simulink model "runsim"  (R2019a)
settings: Solver=VariableStepAuto  StartTime=0.0  StopTime=10.0  RelTol=1e-3
values from neighbouring files (symbols this model uses):
  omega = zeros(N-1,1)    [dubincarminimisevel_venanzio.m]    (also in dubincarminimisevel_venanzio2.m; dubincarminimisevel_venanzio_fine.m; dubincarminimisevel_venanzio_orig.m)
  v = rand(N-1,1)    [DubinsCarMinVel_5varmodel.m]    (also in DubinsCarMinVel_6varmodel.m; DubinsCar_bloatedcode.m = X(:,5); dubincarminimisevel.m = X(:,5); dubincarminimisevel_venanzio.m = ones(N-1,1))
settings Model: Creator=vcichella  LastModifiedBy=Thomas

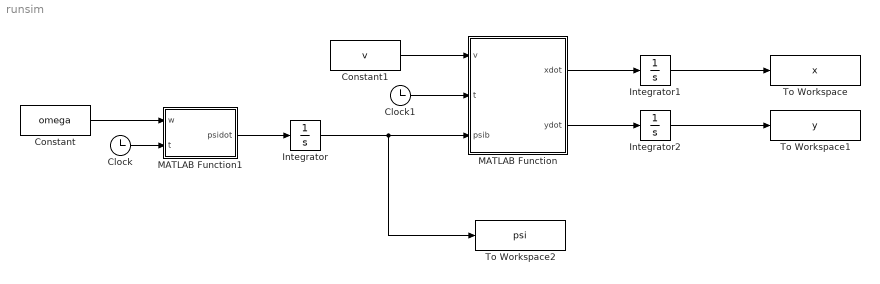
== system runsim ==
  Clock : Clock
  Clock1 : Clock
  Constant : Constant  Value=omega
  Constant1 : Constant  Value=v
  Integrator : Integrator
  Integrator1 : Integrator  InitialCondition=-10
  Integrator2 : Integrator  InitialCondition=40
  MATLAB Function : MATLAB Function  TreatAsAtomicUnit=on
  MATLAB Function1 : MATLAB Function  TreatAsAtomicUnit=on
  To Workspace : ToWorkspace  VariableName=x  SaveFormat=Structure With Time  SampleTime=-1
  To Workspace1 : ToWorkspace  VariableName=y  SaveFormat=Structure With Time  SampleTime=-1
  To Workspace2 : ToWorkspace  VariableName=psi  SaveFormat=Structure With Time  SampleTime=-1
  wires:
  Constant/1 -> MATLAB Function1/1(w)
  Clock/1 -> MATLAB Function1/2(t)
  MATLAB Function1/1(psidot) -> Integrator/1
  Integrator/1 -> To Workspace2/1, MATLAB Function/3(psib)
  Clock1/1 -> MATLAB Function/2(t)
  Constant1/1 -> MATLAB Function/1(v)
  MATLAB Function/1(xdot) -> Integrator1/1
  MATLAB Function/2(ydot) -> Integrator2/1
  Integrator1/1 -> To Workspace/1
  Integrator2/1 -> To Workspace1/1

== matlab function runsim/MATLAB Function1 ==
  data: w input; psidot output; t input
function psidot = fcn(w,t)

T = 10;

coder. extrinsic('BernsteinPoly') 

psidot = 0;

psidot = BernsteinPoly(w',t,0,T);

== matlab function runsim/MATLAB Function ==
  data: v input; t input; xdot output; psib input; ydot output
function [xdot,ydot] = fcn(v,t,psib)

T = 10;

coder.extrinsic('BernsteinPoly') 

vb = BernsteinPoly(v',t,0,T);

xdot = 0;
ydot = 0;

xdot = vb*cos(psib);
ydot = vb*sin(psib);
